simulink model "Contoller_Plant"  (R2020b)
settings: Solver=VariableStepAuto  StartTime=0.0  StopTime=50  RelTol=1e-3
settings Model: Creator=Administrator  LastModifiedBy=Administrator

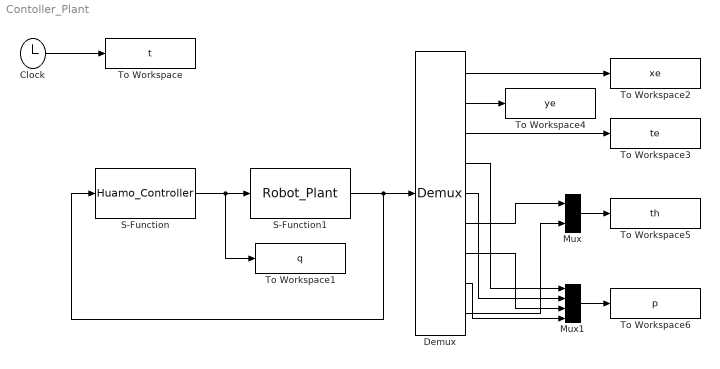
== system Contoller_Plant ==
  Clock : Clock
  Demux : Demux  Outputs=9
  Mux : Mux  Inputs=2
  Mux1 : Mux
  S-Function : S-Function  FunctionName=Huamo_Controller  SFunctionDeploymentMode=off  EnableBusSupport=off
  S-Function1 : S-Function  FunctionName=Robot_Plant  SFunctionDeploymentMode=off  EnableBusSupport=off
  To Workspace : ToWorkspace  VariableName=t  SampleTime=-1
  To Workspace1 : ToWorkspace  VariableName=q  SampleTime=-1
  To Workspace2 : ToWorkspace  VariableName=xe  SaveFormat=Timeseries  SampleTime=-1
  To Workspace3 : ToWorkspace  VariableName=te  SaveFormat=Timeseries  SampleTime=-1
  To Workspace4 : ToWorkspace  VariableName=ye  SaveFormat=Timeseries  SampleTime=-1
  To Workspace5 : ToWorkspace  VariableName=th  SampleTime=-1
  To Workspace6 : ToWorkspace  VariableName=p  SampleTime=-1
  wires:
  Clock/1 -> To Workspace/1
  S-Function/1 -> To Workspace1/1, S-Function1/1
  S-Function1/1 -> S-Function/1, Demux/1
  Demux/2 -> To Workspace4/1
  Demux/1 -> To Workspace2/1
  Demux/3 -> To Workspace3/1
  Mux/1 -> To Workspace5/1
  Mux1/1 -> To Workspace6/1
  Demux/6 -> Mux/1
  Demux/9 -> Mux/2
  Demux/4 -> Mux1/1
  Demux/5 -> Mux1/2
  Demux/7 -> Mux1/3
  Demux/8 -> Mux1/4
